simulink model "ACCELEROMETER"  (R2019b)
settings: Solver=VariableStepAuto  StartTime=0.0  StopTime=10.0  RelTol=1e-3
undefined symbols (not defined in the file): D, K, Kt, M
libraries: simulink x2
settings Model: Creator=simone  LastModifiedBy=simone

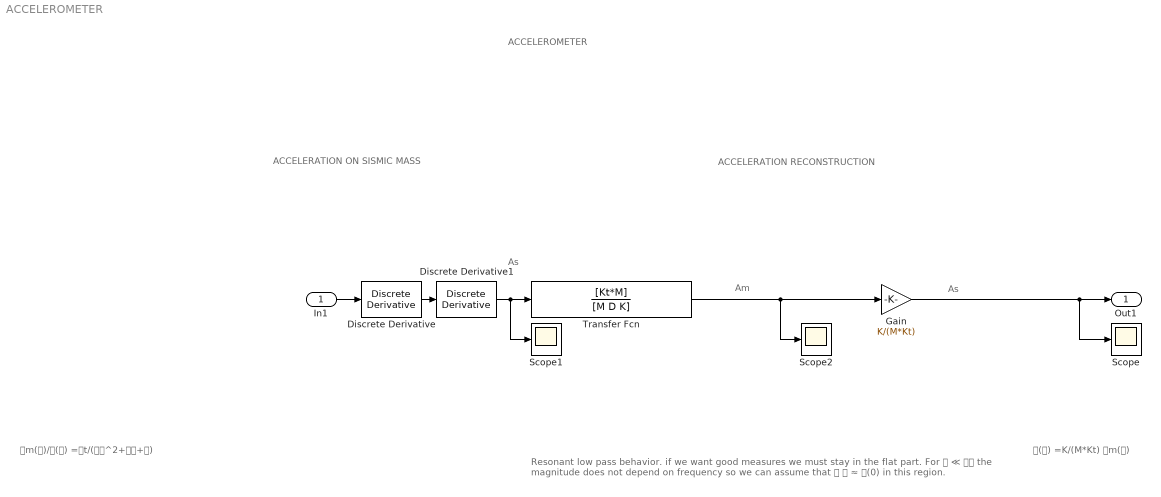
== system ACCELEROMETER ==
  note: ACCELEROMETER
  note: Resonant low pass behavior. if we want good measures we must stay in the flat part.
      | For 𝜔 ≪ 𝜔𝑛 the magnitude does not depend on frequency so we can assume that 𝐺 𝑠 ≈ 𝐺(0) in this region.
  note: Am
  note: As
  note: ACCELERATION RECONSTRUCTION
  note: ACCELERATION ON SISMIC MASS
  note: 𝐴m(𝑠)/𝐴(𝑠) =𝐾t/(𝑀𝑠^2+𝐷𝑠+𝐾)
  note: As
  note: 𝐴(𝑠) =K/(M*Kt) 𝐴m(𝑠)
  In1 : Inport
  Discrete Derivative : simulink/Discrete/Discrete Derivative  gainval=1.0  ICPrevScaledInput=0.0  OutMin=[]  OutMax=[]  OutDataType=fixdt(1, 16)  OutScaling=2^-10  DoSatur=off
  Discrete Derivative1 : simulink/Discrete/Discrete Derivative  gainval=1.0  ICPrevScaledInput=0.0  OutMin=[]  OutMax=[]  OutDataType=fixdt(1, 16)  OutScaling=2^-10  DoSatur=off
  Gain : Gain  Gain=K/(M*Kt)
  Scope : Scope
  Scope1 : Scope
  Scope2 : Scope
  Transfer Fcn : TransferFcn  Numerator=[Kt*M]  Denominator=[M D K]
  Out1 : Outport
  wires:
  In1/1 -> Discrete Derivative/1
  Discrete Derivative/1 -> Discrete Derivative1/1
  Discrete Derivative1/1 -> Transfer Fcn/1, Scope1/1
  Transfer Fcn/1 -> Scope2/1, Gain/1
  Gain/1 -> Scope/1, Out1/1
